simulink model "Vehicle_Model_Controller_Nov16"  (R2020b)
settings: Solver=VariableStepAuto  StartTime=0.0  StopTime=30  FixedStep=0.015  MaxStep=0.1  RelTol=1e-3
model workspace (MAT data in the model file):
  Kp = 10
  understeer_gradient = 0.05
undefined symbols (not defined in the file or in its folder): front_forces, rear_forces
libraries: fl_lib x24, nesl_utility x20, sdl_lib x8, pid_lib x1, vehdynlibsteering x1, autolibshared x1, autolibdatasheetbattery x1
(part 2 of 2)

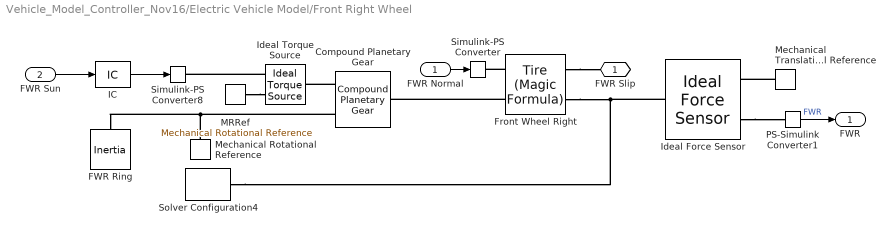
== system Vehicle_Model_Controller_Nov16/Electric Vehicle Model/Front Right Wheel ==
  FWR Normal : Inport
  FWR Sun : Inport  Port=2
  Compound Planetary Gear : sdl_lib/Gears/Compound Planetary Gear  rp_ratio=84/23  ps_ratio=37/24  friction_model=sdl.enum.gear_friction.none  mu_visc=[0, 0] N*m/(rad/s)  efficiency=[.96, .98]  temperature_TLU=[280, 300, 320] K  efficiency_sp_TLU=[.95, .9, .85]  efficiency_rp_TLU=[.95, .9, .85]  pwr_thr=[.001, .001] W  thermal_mass=50 J/K  T_init=300 K  model_inertia=simscape.enum.onoff.off  planet_inertia=0.001 kg*m^2
      settings: SourceProductBaseCode=LD  InternalSimscapePortConfiguration="{\"Bottom\":[],\"Left\":[{\"id\":\"C\",\"label\":\"C\",\"type\":\"foundation.mechanical.rotational.rotational\"}],\"Right\":[{\"id\":\"R\",\"label\":\"R\",\"type\":\"foundation.mechanical.rotational.rotational\"},{\"id\":\"S\",\"label\":\"S\",\"type\":\"foundation.mechanical.rotational.rotational\"}],\"Top\":[]}"
  FWR Ring : fl_lib/Mechanical/Rotational Elements/Inertia  inertia=0.1 kg*m^2  num_ports=foundation.enum.numPorts2.one  w_specify=off  w_priority=High  w=0 rad/s  w_nominal_specify=off  w_nominal_unit=rad/s  w_nominal_value=1  t_specify=off  t_priority=None  t=0 N*m  t_nominal_specify=off  t_nominal_unit=N*m  t_nominal_value=1
  Front Wheel Right : sdl_lib/Tires & Vehicles/Tire (Magic Formula)  parameterization=sdl.enum.magic_tire_model.constant  F_z1=3000 N  F_x1=3500 N  kappa1=10  B_m=10  C_m=1.9  D_m=1.5  E_m=0.97  fz0=4000 N  p_Cx=1.685  p_Dx=[1.21, -.037]  p_Ex=[.344, .095, -.02, 0]  p_Kx=[21.51, -.163, .245]  p_Hx=[-.002, .002]  p_Vx=[0, 0]  v_tr_thr=0.1 m/s  r_e=0.22 m  model_compliance=1  stiffness=2e5 N/m  damping=1000 N/(m/s)  model_inertia=1  inertia=0.03 kg*m^2  initial_velocity=0 rad/s  model_resistance=0  resistance_model=1  coeff=0.015  p_tire=82.74e3 Pa  alpha=-0.003  beta=0.97  coeff_a=84e-4  coeff_b=6.2e-4 s/m  coeff_c=1.6e-4 s^2/m^2  v_thr=0.001 m/s
  IC : InitialCondition  Value=0
  Ideal Force Sensor : fl_lib/Mechanical/Mechanical Sensors/Ideal Force Sensor
  Ideal Torque Source : fl_lib/Mechanical/Mechanical Sources/Ideal Torque Source
      settings: SourceProductName=Foundation Library
  MRRef : fl_lib/Mechanical/Rotational Elements/Mechanical Rotational Reference
      settings: SourceProductName=Foundation Library
  Mechanical Rotational Reference : fl_lib/Mechanical/Rotational Elements/Mechanical Rotational Reference
  Mechanical Translational Reference : fl_lib/Mechanical/Translational Elements/Mechanical Translational Reference
  PS-Simulink Converter1 : nesl_utility/PS-Simulink Converter  PhysicalDomain=network_engine_domain  SubClassName=ps_output  LeftPortType=input  RightPortType=output  PseudoPeriodic=off  Frequencies=[]  Unit=inherit  AffineConversion=off
      settings: SourceProductBaseCode=PW,SS
  Simulink-PS Converter : nesl_utility/Simulink-PS Converter  PhysicalDomain=network_engine_domain  SubClassName=ps_input  LeftPortType=input  RightPortType=output  PseudoPeriodic=off  Frequencies=[]  NoiseDistribution=none  NoiseParameters=[]  Unit=N  AffineConversion=off  FilteringAndDerivatives=zero  SimscapeFilterOrder=1  InputFilterTimeConstant=0.001  UdotUserProvided=0
      settings: SourceProductBaseCode=PW,SS
  Simulink-PS Converter8 : nesl_utility/Simulink-PS Converter  PhysicalDomain=network_engine_domain  SubClassName=ps_input  LeftPortType=input  RightPortType=output  PseudoPeriodic=off  Frequencies=[]  NoiseDistribution=none  NoiseParameters=[]  Unit=N*m  AffineConversion=off  FilteringAndDerivatives=zero  SimscapeFilterOrder=1  InputFilterTimeConstant=0.001  UdotUserProvided=0
      settings: SourceProductBaseCode=PW,SS
  Solver Configuration4 : nesl_utility/Solver Configuration  PhysicalDomain=network_engine_domain  SubClassName=solver  LeftPortType=input  RightPortType=generic  Tones=[]  Harmonics=[]  SimulateNoise=off  Profile=off  UseLocalSampling=off  EnableSwitchedLinearOptims=on  FrequencyDomain=off  UseCCode=off  RelTol=0.001  AbsTol=1e-06  MinStep=1e-09  ToWorkspace=off  RevertToSquareIcSolve=off  NumHomotopyIterations=100  PhasorMode=off  PhasorModeNumHarmonics=1  DoDC=off  ResidualTolerance=1e-09  UseLocalSolver=off  LocalSolverChoice=NE_BACKWARD_EULER_ADVANCER  LocalSolverSampleTime=0.001  DoFixedCost=off  MaxNonlinIter=200  MaxModeIter=20  ComputeImpulses=off  ImpulseIterations=2  LinearAlgebra=auto  EquationFormulation=NE_TIME_EF  DelaysMemoryBudget=1024  AutomaticFiltering=on  FilteringTimeConstant=0.001  PartitionStorageMethod=AS_NEEDED  PartitionMemoryBudget=1024  PartitionMethod=ROBUST
      settings: SourceProductBaseCode=PW,SS
  FWR Slip : PMIOPort  Side=Right
  FWR : Outport
  wires:
  PS-Simulink Converter1/1 -> FWR/1  "FWR"
  FWR Normal/1 -> Simulink-PS Converter/1
  IC/1 -> Simulink-PS Converter8/1
  FWR Sun/1 -> IC/1
  connections:
  Front Wheel Right/RConn1 -- FWR Slip/RConn1
  Front Wheel Right/LConn1 -- Simulink-PS Converter/RConn1
  Ideal Force Sensor/RConn2 -- PS-Simulink Converter1/LConn1
  Ideal Force Sensor/LConn1 -- Front Wheel Right/RConn2 -- Solver Configuration4/RConn1
  Mechanical Translational Reference/LConn1 -- Ideal Force Sensor/RConn1
  MRRef/LConn1 -- Ideal Torque Source/RConn2
  Compound Planetary Gear/RConn2 -- Ideal Torque Source/LConn1
  Ideal Torque Source/RConn1 -- Simulink-PS Converter8/RConn1
  Front Wheel Right/LConn2 -- Compound Planetary Gear/LConn1
  Mechanical Rotational Reference/LConn1 -- FWR Ring/LConn1 -- Compound Planetary Gear/RConn1

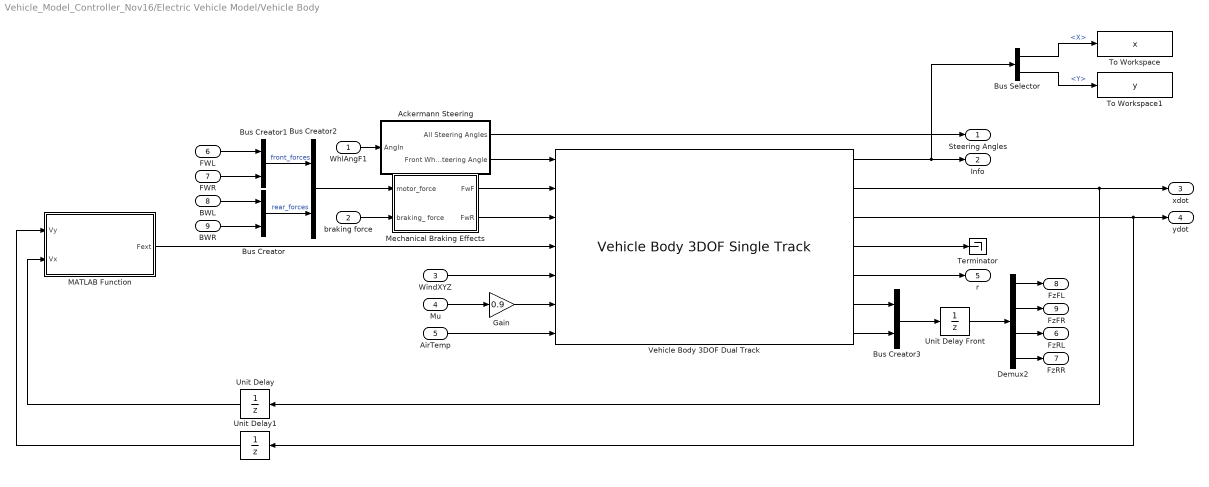
== system Vehicle_Model_Controller_Nov16/Electric Vehicle Model/Vehicle Body ==
  WhlAngF1 : Inport
  braking force : Inport  Port=2
  WindXYZ : Inport  Port=3
  Mu : Inport  Port=4
  AirTemp : Inport  Port=5
  FWL : Inport  Port=6
  FWR : Inport  Port=7
  BWL : Inport  Port=8
  BWR : Inport  Port=9
  Ackermann Steering : Subsystem
  Bus Creator : BusCreator  Inputs=BWL Force,BWR Force
  Bus Creator1 : BusCreator  Inputs=FWL Force,FWR Force
  Bus Creator2 : BusCreator  Inputs=front_forces,rear_forces
  Bus Creator3 : BusCreator  Inputs=2
  Bus Selector : BusSelector  OutputSignals=InertFrm.Cg.Disp.X,InertFrm.Cg.Disp.Y
  Demux2 : Demux
  Gain : Gain  Gain=0.9
  MATLAB Function : MATLAB Function  TreatAsAtomicUnit=on
  Mechanical Braking Effects : Subsystem
  Terminator : Terminator
  To Workspace : ToWorkspace  VariableName=x  SaveFormat=Timeseries  SampleTime=-1
  To Workspace1 : ToWorkspace  VariableName=y  SaveFormat=Timeseries  SampleTime=-1
  Unit Delay : UnitDelay  SampleTime=-1  HasFrameUpgradeWarning=on
  Unit Delay Front : UnitDelay  InitialCondition=[547, 547, 547, 547]  SampleTime=-1  HasFrameUpgradeWarning=on
  Unit Delay1 : UnitDelay  SampleTime=-1  HasFrameUpgradeWarning=on
  Vehicle Body 3DOF Dual Track : autolibshared/Vehicle Body 3DOF Single Track  trackMode=Dual  inputMode=External longitudinal forces  frontSteerMode=on  rearSteerMode=off  windMode=on  muMode=on  extFMode=on  extMMode=off  htchFMode=off  htchMMode=off  extXo=off  extpsio=off  extxdoto=off  extro=off  extYo=off  extTamb=on  extydoto=off  aMode=2  NF=2  NR=2  m=308  a=0.7922471  b=0.7828529  h=0.295  dh=1  hh=0.2  X_o=0  xdot_o=0  CalphaMode=off  sigmaMode=on  d=0  hl=0  w=[1.29579,1.24204]  Cy_f=11e3  Cy_r=11e3  sigma_f=.1  sigma_r=.1  alpha_f_brk=[-.1 .1]  Cy_f_data=[-9e3 9e3]  alpha_r_brk=[-.1 .1]  Cy_r_data=[-9e3 9e3]  Y_o=0  ydot_o=0  Izz=4000  psi_o=0  r_o=0  Af=1.0221  Cd=1.149  Cl=0  Cpm=.000001  beta_w=[0:0.01:0.3]  Cs=[0:0.03:0.9]  Cym=[0:0.01:0.3]  Pabs=101325  Tair=273  g=9.81  mu=1  xdot_tol=.1  Fznom=15000  Fxtire_sat=7e4  Fytire_sat=7e4  longOff=0  latOff=0  vertOff=0  wrapAng=off
      settings: SourceProductBaseCode=PW,DR,MT,UV,VE
  Steering Angles : Outport
  Info : Outport  Port=2
  xdot : Outport  Port=3
  ydot : Outport  Port=4
  r : Outport  Port=5
  FzRL : Outport  Port=6
  FzRR : Outport  Port=7
  FzFL : Outport  Port=8
  FzFR : Outport  Port=9
  wires:
  Vehicle Body 3DOF Dual Track/3 -> Unit Delay1/1, ydot/1
  Mechanical Braking Effects/1(FwF) -> Vehicle Body 3DOF Dual Track/2
  Vehicle Body 3DOF Dual Track/1 -> Info/1, Bus Selector/1
  AirTemp/1 -> Vehicle Body 3DOF Dual Track/7
  Vehicle Body 3DOF Dual Track/4 -> Terminator/1
  Vehicle Body 3DOF Dual Track/5 -> r/1
  Mechanical Braking Effects/2(FwR) -> Vehicle Body 3DOF Dual Track/3
  Ackermann Steering/2(Front Wheels Steering Angle) -> Vehicle Body 3DOF Dual Track/1
  WindXYZ/1 -> Vehicle Body 3DOF Dual Track/5
  Demux2/1 -> FzFL/1
  Demux2/2 -> FzFR/1
  FWL/1 -> Bus Creator1/1
  FWR/1 -> Bus Creator1/2
  Demux2/3 -> FzRL/1
  Demux2/4 -> FzRR/1
  BWL/1 -> Bus Creator/1
  BWR/1 -> Bus Creator/2
  Bus Creator2/1 -> Mechanical Braking Effects/1(motor_force)
  Bus Creator1/1 -> Bus Creator2/1  "front_forces"
  Bus Creator/1 -> Bus Creator2/2  "rear_forces"
  Gain/1 -> Vehicle Body 3DOF Dual Track/6
  Mu/1 -> Gain/1
  Ackermann Steering/1(All Steering Angles) -> Steering Angles/1
  WhlAngF1/1 -> Ackermann Steering/1(AngIn)
  Bus Selector/1 -> To Workspace/1  "<X>"
  Bus Selector/2 -> To Workspace1/1  "<Y>"
  Vehicle Body 3DOF Dual Track/7 -> Bus Creator3/2
  Vehicle Body 3DOF Dual Track/6 -> Bus Creator3/1
  Bus Creator3/1 -> Unit Delay Front/1
  Unit Delay Front/1 -> Demux2/1
  MATLAB Function/1(Fext) -> Vehicle Body 3DOF Dual Track/4
  Unit Delay/1 -> MATLAB Function/2(Vx)
  Unit Delay1/1 -> MATLAB Function/1(Vy)
  braking force/1 -> Mechanical Braking Effects/2(braking_	force)
  Vehicle Body 3DOF Dual Track/2 -> xdot/1, Unit Delay/1

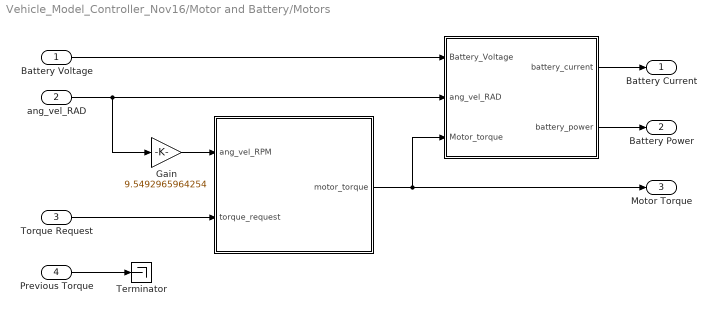
== system Vehicle_Model_Controller_Nov16/Motor and Battery/Motors ==
  Battery Voltage : Inport
  ang_vel_RAD : Inport  Port=2
  Torque Request : Inport  Port=3
  Previous Torque : Inport  Port=4
  " " : MATLAB Function  TreatAsAtomicUnit=on
  "  " : MATLAB Function  TreatAsAtomicUnit=on
  Gain : Gain  Gain=9.5492965964254
  Terminator : Terminator
  Battery Current : Outport
  Battery Power : Outport  Port=2
  Motor Torque : Outport  Port=3
  wires:
  Torque Request/1 -> " "/2(torque_request)
  Battery Voltage/1 -> "  "/1(Battery_Voltage)
  ang_vel_RAD/1 -> Gain/1, "  "/2(ang_vel_RAD)
  "  "/1(battery_current) -> Battery Current/1
  " "/1(motor_torque) -> Motor Torque/1, "  "/3(Motor_torque)
  "  "/2(battery_power) -> Battery Power/1
  Gain/1 -> " "/1(ang_vel_RPM)
  Previous Torque/1 -> Terminator/1

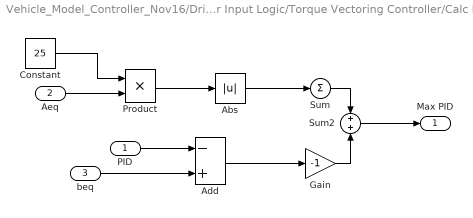
== system Vehicle_Model_Controller_Nov16/Driver Input Logic/Torque Vectoring Controller/Calc Max PID ==
  PID : Inport
  Aeq : Inport  Port=2
  beq : Inport  Port=3
  Abs : Abs
  Add : Sum  Inputs=-+
  Constant : Constant  Value=25
  Gain : Gain  Gain=-1
  Product : Product
  Sum : Sum  Inputs=1
  Sum2 : Sum
  Max PID : Outport
  wires:
  Add/1 -> Gain/1
  Product/1 -> Abs/1
  PID/1 -> Add/1
  Abs/1 -> Sum/1
  Sum2/1 -> Max PID/1
  Gain/1 -> Sum2/2
  Sum/1 -> Sum2/1
  Aeq/1 -> Product/2
  Constant/1 -> Product/1
  beq/1 -> Add/2

== system Vehicle_Model_Controller_Nov16/Driver Input Logic/Torque Vectoring Controller/Calc Power Consumption ==
  Required Torque : Inport
  Motor Shaft Velocity : Inport  Port=2
  Product : Product
  Sum : Sum  Inputs=|+
  Transpose : Math  Operator=transpose  SaturateOnIntegerOverflow=on
  Power : Outport
  wires:
  Product/1 -> Sum/1
  Motor Shaft Velocity/1 -> Transpose/1
  Transpose/1 -> Product/2
  Required Torque/1 -> Product/1
  Sum/1 -> Power/1

== system Vehicle_Model_Controller_Nov16/Electric Vehicle Model/Vehicle Body/Ackermann Steering ==
  AngIn : Inport
  Bus Creator : BusCreator  Inputs=2
  Deg to Rad : Gain  Gain=pi/180
  Kinematic Steering : vehdynlibsteering/Kinematic Steering  StrgType=Ackerman  StrgRatioType=Constant  Loc=Front  NrmlFctr=1  TrckWdth=1.29579  WhlBase=1.5751  Db=0  StrgRng=1.25*pi  StrgAngBpts="[-6.2832   -5.0265   -3.7699   -2.5133   -1.2566         0    1.2566    2.5133    3.7699    5.0265    6.2832]"  StrgRatioTbl=|  StrgRatio=1  StrgArmLngth=0.1  RckCsLngth=0.5  TieRodLngth=0.248  D=0.2  PnnRadius=0.0057  PnnRadiusTbl="[0.0055    0.0055    0.0056    0.0057    0.0058    0.0057    0.0057    0.0057    0.0056    0.0055    0.0055]"  RodLngth=0.1  ParaArmLngth=0.9  aMode=2
      | [13.5000   13.3750   13.2500   13.1250   13.0000   13.0000   13.0000   13.1250   13.2500   13.3750   13.5000
      | ]
  Mux3 : Mux  Inputs=2
  Terminator : Terminator
  All Steering Angles : Outport
  Front Wheels Steering Angle : Outport  Port=2
  wires:
  Kinematic Steering/2 -> Mux3/1
  Kinematic Steering/3 -> Mux3/2
  Kinematic Steering/1 -> Terminator/1
  Mux3/1 -> Front Wheels Steering Angle/1, Bus Creator/1  "ackermann angles"
  Bus Creator/1 -> All Steering Angles/1
  Deg to Rad/1 -> Kinematic Steering/1, Bus Creator/2  "steering_angle"
  AngIn/1 -> Deg to Rad/1  "steering_angle"

== system Vehicle_Model_Controller_Nov16/Electric Vehicle Model/Vehicle Body/Mechanical Braking Effects ==
  motor_force : Inport
  braking_	force : Inport  Port=2
  Bus Selector : BusSelector  OutputSignals=front_forces,rear_forces
  mechanical_braking_effects : MATLAB Function  TreatAsAtomicUnit=on
  FwF : Outport
  FwR : Outport  Port=2
  wires:
  mechanical_braking_effects/1(FwF) -> FwF/1
  braking_	force/1 -> mechanical_braking_effects/1(braking_forces)
  mechanical_braking_effects/2(FwR) -> FwR/1
  Bus Selector/1 -> mechanical_braking_effects/2(front_forces)  "<front_forces>"
  Bus Selector/2 -> mechanical_braking_effects/3(rear_forces)  "<rear_forces>"
  motor_force/1 -> Bus Selector/1

== matlab function Vehicle_Model_Controller_Nov16/Driver Input Logic/Torque Vectoring Controller/Layer 2 ==
  data: prev_torque input; yaw_err output; prev_torque output; J_z output; T2F input; P_L input; eff_m input; s input; yaw_ref input; yaw input; J_z input; l input; a_theta input; c_theta input; driver_input input; P input; vel input; Fy input; gr input; r input; F_max input; y output; x output; Fy_wheel output; driver_input output; P_C output; eff_m output; T2F output; slip_limit output; power_limit output; omega_m output size=[1 4]; t_upper output; tau input; t_minmax input; t_lower output; f input; t_minmax output; brake_force input
function [yaw_err, prev_torque, J_z, y, x, Fy_wheel, driver_input, P_C, eff_m, T2F, slip_limit, power_limit, omega_m, t_upper, t_lower, t_minmax] = Layer_2(prev_torque, T2F, P_L, eff_m, s, yaw_ref, yaw, J_z, l, a_theta, c_theta, driver_input, P, vel, Fy, gr, r, F_max, tau, t_minmax, f, brake_force)
%% Calculations
% Calculate the Yaw Error, Apply Sign Convention
if yaw_ref(1) == 0 && yaw(1) == 0
    yaw_err = 0;
elseif c_theta >= 0
    yaw_err = min(abs(yaw_ref)) - yaw;
else
    yaw_err = (min(abs(yaw_ref)) * -1) - yaw;
end


% Motor Shaft Speed, RAD/S
omega_fl = (vel(1) * cos(a_theta(1))) + (vel(2) * sin(a_theta(1)));
omega_fr = (vel(3) * cos(a_theta(2))) + (vel(4) * sin(a_theta(2)));
omega_rl = vel(5);
omega_rr = vel(6);

omega_m = [omega_fl, omega_fr, omega_rl, omega_rr] .* (gr ./ r);


% Calculate K_1 Vehicle Constants
x_1 = (s(1) * cos(a_theta(1))) + (l(1) * sin(a_theta(1)));    
x_2 = (-1 * s(1) * cos(a_theta(2))) + (l(1) * sin(a_theta(2)));     
x_3 = s(2);     
x_4 = -s(2); 

x = [x_1, x_2, x_3, x_4]; 


% Transform Lateral Forces (Vehicle) to Lateral Forces (Wheel)
F_y_ij_fl = (sin(a_theta(1)) * Fy(1)) + (cos(a_theta(1)) * Fy(1));
F_y_ij_fr = (sin(a_theta(2)) * Fy(2)) + (cos(a_theta(2)) * Fy(2));
F_y_ij_rl = Fy(3);
F_y_ij_rr = Fy(4);

Fy_wheel = [F_y_ij_fl, F_y_ij_fr, F_y_ij_rl, F_y_ij_rr];


% Calculate K_2 Vehicle Constants
y_1 = (-1 * s(1) * sin(a_theta(1))) + (l(1) * cos(a_theta(1)));    
y_2 = (s(1) * sin(a_theta(2))) + (l(1) * cos(a_theta(2)));
y_3 = -l(2);
y_4 = -l(2);

y = [y_1, y_2, y_3, y_4]; 


% Longitudinal force Limits On Individual Wheels
Fx_max2 = (F_max.^2)-(Fy_wheel.^2);

% Control For Negative Output
for i = 1:4
    if Fx_max2(i) < 0
        Fx_max2(i) = 0;
    end
end

% Calculate Torque Limit Due to Power and Slip
Fx_max = sqrt(Fx_max2)-brake_force;
slip_limit = Fx_max ./ T2F; 
power_limit = (P_L .* eff_m) ./ omega_m;


% Erase power limit solution above torque limit, for better data
% visualization
for i = 1:4
    if power_limit(i) > 25 
        power_limit(i) = 25;
    elseif power_limit(i) < -25
        power_limit(i) = -0.01; 
    end
end 

% Calculate Constants for getting limit on motor output torque
e_term = exp(-1 / (tau * f));
c_lower = (1 - e_term) .* t_minmax(1);
c_upper = (1 - e_term) .* t_minmax(2);
c_constant = (prev_torque .* e_term)';

% Max and Min Torque Limits
t_upper = max([c_upper + c_constant; c_constant + .01]);
t_lower = min([c_lower + c_constant; c_constant - .01]);

% If driver is not pressing acceleration pedal, no positive torque is allowed
if driver_input <= 0
   t_upper = [0, 0, 0, 0];
   P_C = P(2);  
else
    P_C = P(1);
end


end

== matlab function Vehicle_Model_Controller_Nov16/Electric Vehicle Model/Vehicle Body/MATLAB Function ==
  data: Vy input; Vx input; Fext output
function Fext = get_downforce(Vy, Vx)
%% Constants
rho = 1.225; % Air density [Kg/m^3]
cl = 2.11014; % Lift coefficient [unitless]
A = 1.0221; % Frontal Area [m^2]


%% Computation
% Compute CoG Velocity
Vcog = Vx^2 + Vy^2;

% Compute DownForce
Fz = 0.5 * rho * Vcog * cl * A;
Fext = [0, 0, Fz];

== matlab function Vehicle_Model_Controller_Nov16/Motor and Battery/Motors/  ==
  data: ang_vel_RPM input; motor_torque output size=[1 4]; torque_request input
function motor_torque = get_torque(ang_vel_RPM, torque_request)
%% Actual Torque Output
% Developers:    Demetrius Gulewicz

% Developed for: Purdue Electric Racing
% Date:          09/18/2021
%
% Definitions:
% ang_vel:   Angular velocity of each wheel on the wheel fixed y axis [RPM]
% torque_request: Requested torque from the LP model                  [Nm]

%% Constants
% quadratic constants that connect current and max RPM of motors
a_v = 0.2667;
b_v = -66.353;
c_v = 10452 - ang_vel_RPM;

% quadratic constants that connnect current and max torque of motors
a_t = -0.0987;
b_t = 45.799;
c_t = -129.65;

% maximum possible current at the current RPM
max_current = [0, 0, 0, 0];


%% Calculate Maximum Torque Possible
% calculate the maximum current possible at the current RPM
for i = [1:4]
   if ang_vel_RPM(i) < 7000
       max_current(i) = 70;
   else
       max_current(i) = (-b_v - sqrt(b_v^2 - (4*a_v.*c_v(i)))) .* (1/(2*a_v));
   end
end

% calculate the meximum torque at the max current
max_torque = (a_t .* (max_current.^2)) + (b_t .* max_current) + c_t;
for i = [1:4]
   if max_torque(i) < 0
      max_torque(i) = 0;
   end
end

motor_torque_matrix = [max_torque; torque_request'];
motor_torque = min(motor_torque_matrix);

== matlab function Vehicle_Model_Controller_Nov16/Electric Vehicle Model/Vehicle Body/Mechanical Braking Effects/mechanical_braking_effects ==
  data: braking_forces input; front_forces input; FwF output; rear_forces input; FwR output
function [FwF, FwR] = Mechanical_Braking_Effects(braking_forces, front_forces, rear_forces)
%% Mechanical Braking Effects
% Developers:    Demetrius Gulewicz
% Developed for: Purdue Electric Racing
% Date:          09/01/2021
%
% Definitions:
% front_force:      force vector from the front motors    [N]
% braking_forces:   braking force vector on all 4 tires   [N]
% rear_forces:      force vector from the rear motors     [N]

%% Calculation
FwF = front_forces + braking_forces(1:2);
FwR = rear_forces + braking_forces(3:4);

== matlab function Vehicle_Model_Controller_Nov16/Driver Input Logic/MATLAB Function ==
  data: T_brake_trans output; F_brake_trans output; driver_input input; F_brake output; BrakeRatio_Motor output; Vx input
function [T_brake_trans,F_brake_trans,F_brake,BrakeRatio_Motor]= brakeforce(driver_input, Vx)
%% Actual Mechanical Brake Force and Torque Calculation 
% Developer(s):    Tao Sun

% Developed for: Purdue Electric Racing
% Date:          10/26/2021
%
%Parameters:
% brakeforce_max: Maximum cliper force to hold the disk.                 [N]
% brakefriction_coefficent: Friction coefficient between disk and clipper
% disk_diameter: disk diameter                                           [m]


%% Calculation
brakeforce_max = [100,100,100,100]; % [fl fr bl br]
brakefriction_coefficient = [.5,.5,.5,.5]; 
disk_diameter = [0.1,0.1,0.1,0.1]; % in meter
if driver_input >= -0.5            % for small brakes (input >= -0.5), mechanical brake will not work
   brake_torque = [0,0,0,0];
   if driver_input < 0             % BrakeRatio_Motor is the portion of power demanded for motors to produce negative 
                                   % torque. This variable is trnasfered to
                                   % Optimization model to determine power. 
                                      
       BrakeRatio_Motor = driver_input/(-0.5);  % in scale of [0,1]
   else
       BrakeRatio_Motor = 0;
   end
elseif driver_input >=-1           % mechanical brake start to work if driver_input <= -0.5
    % note the actual force may not be proportional to the input. need to discuss with brake team 
    brakeforce_coefficient = [-driver_input/0.5,-driver_input/0.5,-driver_input/0.5,-driver_input/0.5];
    brakeforce_normal = brakeforce_coefficient.*brakeforce_max;
    brake_torque = -1.*brakeforce_normal.*brakefriction_coefficient.*disk_diameter;
    BrakeRatio_Motor = 1;
else
    brake_torque = brakeforce_max.*disk_diameter;  % if driver_input less than -1, full brake
    BrakeRatio_Motor = 1;
end

if Vx > 0
    T_brake = brake_torque * sqrt(abs(Vx));
    F_brake = T_brake./disk_diameter;
    T_brake_trans = T_brake';
    F_brake_trans = F_brake';
else
    T_brake = -brake_torque * sqrt(abs(Vx));
    F_brake = -T_brake./disk_diameter;
    T_brake_trans = -T_brake';
    F_brake_trans = -F_brake';
end

== matlab function Vehicle_Model_Controller_Nov16/Driver Input Logic/Torque Vectoring Controller/LP_Calc  ==
  data: Tx output size=[4 1]; omega_m output; lb output double; PID input; prev_torque input; J_z input; y input; x input; Fy_wheel input; driver_input input; P_C input; eff_m input; T2F input; slip_limit input; power_limit input; omega_m input; t_upper input; ub output double; Aeq output double; beq output double; A output; b output; t_lower input; t_minmax input; BrakeRatio_Motor input; M_max output
function [Tx, omega_m, lb, ub, Aeq, beq, A, b, M_max] = LP_calc(PID, prev_torque, J_z, y, x, Fy_wheel, driver_input, P_C, eff_m, T2F, slip_limit, power_limit, omega_m, t_upper, t_lower, t_minmax,BrakeRatio_Motor)
%% Calculation
% Calculate Boundary Conditions
ub = [0, 0, 0, 0];
lb = [0, 0, 0, 0];

for i = 1:4
    ub(i) = min([slip_limit(i), power_limit(i), t_minmax(2), t_upper(i)]);
    lb(i) = max([-slip_limit(i), -power_limit(i), t_minmax(1), t_lower(i)]);
end

% Enforce no backwards rotation
for i = 1:4
   if omega_m(i) < 240 && lb(i) < -0.1
       lb(i) = -0.001;
   end
end

% Lower & Upper Boundary Forces on the Tires
ub_f = ub .* T2F;
lb_f = lb .* T2F;

% Find Boundaries for PID, the yaw acceleration of the car
M_max=zeros(1,2);
M_max(1) = (x(1)*ub_f(1)+x(3)*ub_f(3)+x(2)*lb_f(2)+x(4)*lb_f(4)+sum(y.*Fy_wheel))/J_z;
M_max(2) = (x(2)*ub_f(2)+x(4)*ub_f(4)+x(1)*lb_f(1)+x(3)*lb_f(3)+sum(y.*Fy_wheel))/J_z;

if PID >= M_max(1)
    PID = M_max(1);
elseif PID <= M_max(2)
    PID = M_max(2);
end

% Calculate Yaw Constraint
Aeq = ((1 ./ J_z) .* x) .* T2F;
beq = PID-sum(((1 / J_z) * y) .* Fy_wheel);

% Calculate Power Constraint
if driver_input >=0
    A = omega_m ./ eff_m;
    b = driver_input*P_C;
else 
    A = -omega_m ./ eff_m;
    b = -BrakeRatio_Motor*P_C;
end


%% Optimization
% Set Optimization Parameters
options = optimoptions('fmincon','Algorithm','sqp');

% Determine correct objective function maximize the forces acting on the car
if driver_input >= 0
    objfun = @(q) -sum(q .* T2F);
    Tx = fmincon(objfun,prev_torque',A,b,Aeq,beq,lb,ub,[],options)';
else 
    objfun = @(q) sum(q .* T2F);    
    Tx = fmincon(objfun,prev_torque',A,b,Aeq,beq,lb,ub,[],options)';
end 

end

== matlab function Vehicle_Model_Controller_Nov16/Motor and Battery/Motors/   ==
  data: Battery_Voltage input; ang_vel_RAD input; battery_current output; Motor_torque input; battery_power output
function [battery_current, battery_power]= get_batt_curr(Battery_Voltage, ang_vel_RAD, Motor_torque)
%% Current Draw
% Developers:    Demetrius Gulewicz

% Developed for: Purdue Electric Racing
% Date:          09/18/2021
%
% Definitions:
% ang_vel_RAD:   Angular velocity of each wheel on the wheel fixed y axis [RAD]
% Motor_torque:  Torque the motor actually outputs                 [Ncm]
% Battery_Voltage: The voltage of the battery                      [V]

%% Definitions
a = 0.0411;
b = 2.7976;
c = 45.978;

t = Motor_torque;
w = ang_vel_RAD;
v = Battery_Voltage;

e = 85;

%% Calculate Current Draw
%x0 = [20, 20, 20, 20];
%options = optimoptions('fsolve','Algorithm','Levenberg-Marquardt');
%F = @(x) ([(a * x(1)^3) + (b * x(1)^2) + (c * x(1)), ] .* v) - (t .* w);
%battery_current = sum(fsolve(F,x0,options));

battery_current = sum((t .* w') ./ (e .* v));
battery_power = battery_current * Battery_Voltage;
end

== matlab function Vehicle_Model_Controller_Nov16/Driver Input Logic/Torque Vectoring Controller/Constants  ==
  data: P_L output; eff_m output; mu output; g output; r output; s output; l output; J_z output; K_u output; gr output; eff_g output; tau output; t_minmax output; f output; c_factor output
function [P_L, eff_m, mu, g, r, s, l, J_z, K_u, gr, eff_g, tau, t_minmax, f, c_factor] = def_constants()
%% Define Constants
% General Constants
mu = [0.8, 0.8, 0.8, 0.8]; % Maximum friction coefficient [Unitless]
g = 9.81; % Gravitational constant [m/s^2]
f = 1 / 0.015; % controller frequency [Hz]
c_factor = 0.8; % Max yaw equation contributing factor [Unitless]

% Motor Constants
P_L = [15, 15, 15, 15] * 1000; % Power limit for each motor [W] 
eff_m = [0.85, 0.85, 0.85, 0.85]; % Motor efficiency [Unitless]
tau = 0.29; % Motor Response Time Constant
t_minmax = [-20, 20]; % Minimum and maximum torque you can request from motor

% General Vehicle Constants
r = 0.22; % Tire radius [m]
s = [0.647895, 0.62102]; % Half track width [m]
l = [0.7922471, 0.7828529]; % Wheelbase [m]
J_z = 4000; % Polar moment of inertia [kg m^2]
K_u = 0.05; % Understeer gradient

% Gearbox Constants
GR_f = (37/24) * (84/23) + 1; % Front gear ratio [Unitless]
GR_r = (40/21) * (84/23) + 1; % Rear gear ratio [Unitless]
gr = [GR_f, GR_f, GR_r, GR_r]; % Gear ratios [Unitless]
eff_g = 0.97; % Gearbox power transmission efficiency [Unitless]


end

== matlab function Vehicle_Model_Controller_Nov16/Driver Input Logic/Torque Vectoring Controller/Layer 1 ==
  data: T2F output; P_L output; eff_m output; s output; yaw_ref output; yaw output; J_z output; l output; a_theta output; c_theta output; driver_input output; P output; vel output; Fy output; gr output; r output; F_max output; P_L input; eff_m input; mu input; g input; r input; s input; l input; J_z input; K_u input; gr input; eff_g input; tau input; t_minmax input; f input; c_factor input; driver_input input; P input; c_theta input; a_theta input; Fx input; Fy input; Fz input; Vx input; Vy input; yaw input; vel input; tau output; t_minmax output; f output
function [T2F, P_L, eff_m, s, yaw_ref, yaw, J_z, l, a_theta, c_theta, driver_input, P, vel, Fy, gr, r, F_max, tau, t_minmax, f] = Layer_1(P_L, eff_m, mu, g, r, s, l, J_z, K_u, gr, eff_g, tau, t_minmax, f, c_factor,driver_input, P, c_theta, a_theta, Fx, Fy, Fz, Vx, Vy, yaw, vel)
%% Calculation
% Max Allowed Force On Each Wheel
F_max = abs(mu'.*Fz)';

% Convert coeffecient to convert Torque At The Motor Shaft to Force At The Wheel
T2F = (gr .* eff_g) ./ r;


% Yaw Calculations
v_cog = sqrt(Vx^2 + Vy^2);
yaw_des = (v_cog * abs(c_theta)) / ((l(1) + l(2)) + (K_u * v_cog ^ 2));
yaw_max = (c_factor * max(mu) * g) / (v_cog);

% control for large max yaw, for better viewing
if yaw_max > 1
    yaw_max = 1;
end

yaw_ref = [yaw_des, yaw_max];

end
